simulink model "RCAMSimulation"  (R2021a)
settings: Solver=VariableStepAuto  StartTime=0.0  StopTime=TF  RelTol=1e-3
values from neighbouring files (symbols this model uses):
  x0 = [85 ... (first row only)    [initializeConstants.m]
undefined symbols (not defined in the file or in its folder): RCAM_model
settings Model: Creator=Hp  LastModifiedBy=Hp

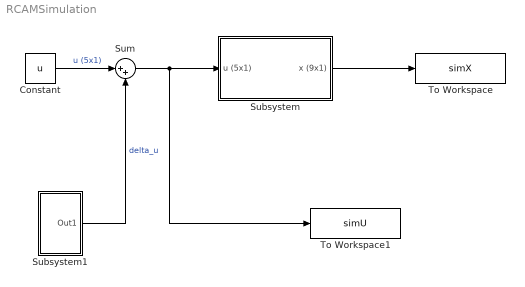
== system RCAMSimulation ==
  Constant : Constant  Value=u
  Subsystem : Subsystem
  Subsystem1 : Subsystem
  Sum : Sum  Inputs=|++
  To Workspace : ToWorkspace  VariableName=simX  SaveFormat=Timeseries  SampleTime=-1
  To Workspace1 : ToWorkspace  VariableName=simU  SaveFormat=Timeseries  SampleTime=-1
  wires:
  Subsystem/1(x (9x1)) -> To Workspace/1
  Constant/1 -> Sum/1  "u (5x1)"
  Subsystem1/1(Out1) -> Sum/2  "delta_u"
  Sum/1 -> To Workspace1/1, Subsystem/1(u (5x1))

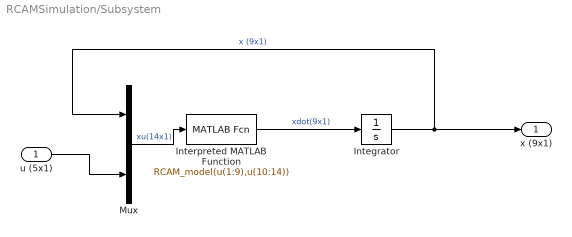
== system RCAMSimulation/Subsystem ==
  u (5x1) : Inport
  Integrator : Integrator  InitialCondition=x0
  Interpreted MATLAB Function : MATLABFcn  MATLABFcn=RCAM_model(u(1:9),u(10:14))
  Mux : Mux  Inputs=2
  x (9x1) : Outport
  wires:
  Interpreted MATLAB Function/1 -> Integrator/1  "xdot(9x1)"
  u (5x1)/1 -> Mux/2
  Integrator/1 -> x (9x1)/1, Mux/1  "x (9x1)"
  Mux/1 -> Interpreted MATLAB Function/1  "xu(14x1)"

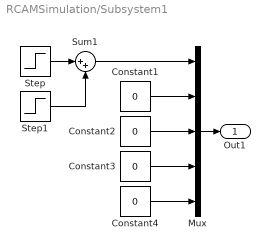
== system RCAMSimulation/Subsystem1 ==
  Constant{1..4} (4 alike) : Constant  Value=0
  Mux : Mux  Inputs=5
  Step : Step  Time=30  After=5*pi/180  SampleTime=0
  Step1 : Step  Time=32  After=-5*pi/180  SampleTime=0
  Sum1 : Sum  Inputs=|++
  Out1 : Outport
  wires:
  Mux/1 -> Out1/1
  Step1/1 -> Sum1/2
  Sum1/1 -> Mux/1
  Constant3/1 -> Mux/4
  Constant1/1 -> Mux/2
  Constant2/1 -> Mux/3
  Constant4/1 -> Mux/5
  Step/1 -> Sum1/1
